simulink model "simulink_experiments_LQ_kal"  (R2019b)
settings: Solver=ode1  StartTime=0.0  StopTime=inf  FixedStep=0.002  RelTol=1e-3  EnableMultiTasking=on
PostLoadFcn:
  | qc_set_target_type(getConfigSet(bdroot, 'QUARC Default Target Configuration'));
undefined symbols (not defined in the file): HIL, kalmf, Klqi_int, Klqi_state, qc_get_step_size
libraries: quarc_library x4
settings Model: SimulationMode=external  ExtModeTrigDuration=5000  Creator=CFulford  LastModifiedBy=Student
settings SolverCC: PositivePriorityOrder=on
settings DataIOCC: LimitDataPoints=on  SaveFormat=Array  SignalLoggingSaveFormat=ModelDataLogs  ReturnWorkspaceOutputs=off
settings OptimizationCC: ExpressionDepthLimit=2147483647  InitFltsAndDblsToZero=on  LifeSpan=inf
settings DebuggingCC: SaveWithParameterizedLinksMsg=none  UnderspecifiedInitializationDetection=Classic  MergeDetectMultiDrivingBlocksExec=none  SolverPrmCheckMsg=warning  MultiTaskDSMMsg=warning  MultiTaskCondExecSysMsg=none  FcnCallInpInsideContextMsg=warning  StateNameClashWarn=warning  SFUnexpectedBacktrackingDiag=warning  SFNoUnconditionalDefaultTransitionDiag=warning  SFExecutionAtInitializationDiag=none  ArithmeticOperatorsInVariantConditions=warning
settings HardwareCC: ProdBitPerPointer=32  ProdBitPerSizeT=32  ProdBitPerPtrDiffT=32  ProdLargestAtomicFloat=None  ProdIntDivRoundTo=Undefined  ProdEndianess=Unspecified  ProdWordSize=32  ProdHWDeviceType=32-bit Generic
settings ModelReferenceCC: PropagateSignalLabelsOutOfModel=off
settings SFSimCC: SimUseLocalCustomCode=off  CustomCodeUndefinedFunction=UseInterfaceOnly
settings RTWCC: Description=QUARC Win64 Target  SystemTargetFile=quarc_win64.tlc  TemplateMakefile=quarc_default_tmf  RTWUseLocalCustomCode=off
settings CodeAppCC: StateflowObjectComments=on
settings STFCustomTargetCC: TargetPreCompLibLocation=C:\PROGRA~3\QUARC\lib\2019b\win64\release  ConcurrentExecutionCompliant=on  GeneratePreprocessorConditionals=Disable all  CombineOutputUpdateFcns=on  CPPClassGenCompliant=on  SystemTargetFile=quarc_win64.tlc
settings GRTTargetCC: TargetPreCompLibLocation=C:\PROGRA~3\QUARC\lib\2019b\win64\release  TargetLangStandard=C89/C90 (ANSI)  ParMdlRefBuildCompliant=off  CompOptLevelCompliant=off  GeneratePreprocessorConditionals=Disable all  MatFileLogging=off  UseToolchainInfoCompliant=off  ExtMode=on  ExtModeMexFile=quarc_comm
settings ConfigComp: CovMetricSettings=dw  CovHtmlReporting=on  CovSaveCumulativeToWorkspaceVar=on  CovSaveSingleToWorkspaceVar=on  CovExternalEMLEnable=off  CovSFcnEnable=off

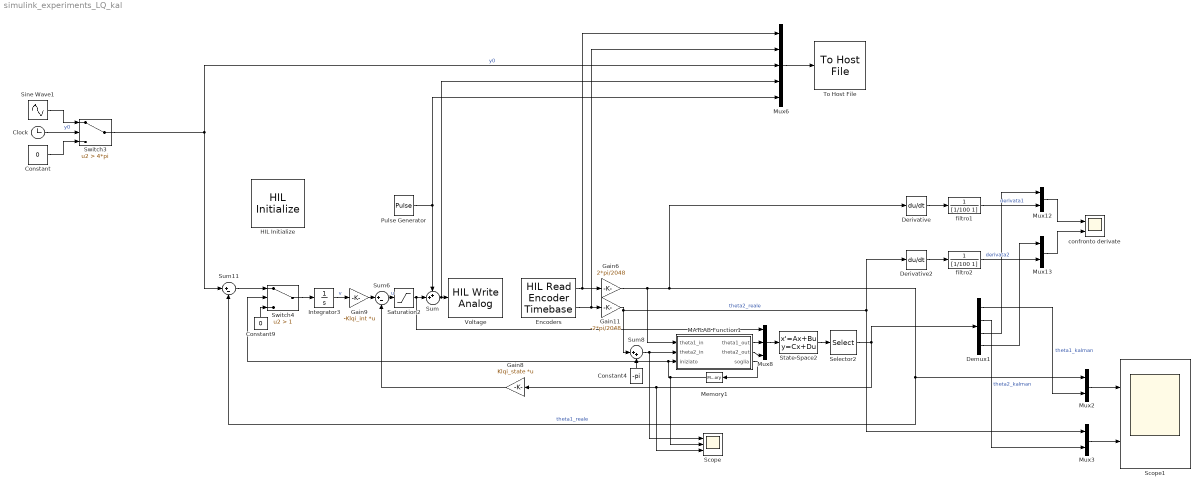
== system simulink_experiments_LQ_kal ==
  Clock : Clock
  Constant : Constant  Value=0
  Constant4 : Constant  Value=-pi
  Constant9 : Constant  Value=0
  Demux1 : Demux
  Derivative : Derivative
  Derivative2 : Derivative
  Encoders : quarc_library/Data Acquisition/Generic/Timebases/HIL Read Encoder Timebase  object_name=HIL-1  clock=0  channels=[0:1]  samples_in_buffer=max(ceil(1/qc_get_step_size), 1)  active=on  vector_output=off  data_type_mode=Inherit via back propagation  data_type=double
  Gain11 : Gain  Gain=-2*pi/2048
  Gain6 : Gain  Gain=2*pi/2048
  Gain8 : Gain  Gain=Klqi_state  Multiplication=Matrix(K*u)
  Gain9 : Gain  Gain=-Klqi_int  Multiplication=Matrix(K*u)
  HIL Initialize : quarc_library/Data Acquisition/Generic/Configuration/HIL Initialize  Priority=-99  object_name=HIL-1  board_type=qube_servo2_usb  board_number=0  board_options=""  exclusive=off  active=off  hardware_clocks=[0]  clock_modes=[]  initial_clock_frequencies=[]  set_clock_params_at_start=off  set_clock_params_at_switch_in=off  set_clock_frequencies_at_start=off  set_clock_frequencies_at_switch_in=off  analog_input_channels=[0]  analog_input_configurations=[]  analog_input_maximums=3  analog_input_minimums=-3  set_analog_input_params_at_start=off  set_analog_input_params_at_switch_in=off  analog_output_channels=[0]  analog_output_maximums=15  analog_output_minimums=-15  initial_analog_outputs=[0]  final_analog_outputs=[0]  watchdog_analog_outputs=0  set_analog_output_params_at_start=off  set_analog_output_params_at_switch_in=off  set_analog_outputs_at_start=on  set_analog_outputs_at_switch_in=off  set_analog_outputs_at_terminate=on  set_analog_outputs_at_switch_out=off  set_analog_outputs_on_watchdog=on  digital_input_channels=[]  digital_output_channels=[0]  digital_output_configuration=[]  initial_digital_outputs=[1]  final_digital_outputs=[0]  watchdog_digital_outputs=[0]  set_digital_output_params_at_start=off  set_digital_output_params_at_switch_in=off  set_digital_outputs_at_start=on  set_digital_outputs_at_switch_in=off  set_digital_outputs_at_terminate=on  set_digital_outputs_at_switch_out=off  set_digital_outputs_on_watchdog=on  encoder_channels=[0:1]  quadrature=[4]  encoder_filter_frequency=[]  initial_encoder_counts=[0]  set_encoder_params_at_start=off  set_encoder_params_at_switch_in=off  set_encoder_counts_at_start=on  set_encoder_counts_at_switch_in=off  pwm_channels=[]  pwm_modes=[]  pwm_frequency=[]  pwm_configuration=[]  pwm_alignment=[]  pwm_polarity=[]  pwm_leading_deadband=[]  pwm_trailing_deadband=[]  initial_pwm_outputs=[]  final_pwm_outputs=[]  watchdog_pwm_outputs=[]  set_pwm_params_at_start=off  set_pwm_params_at_switch_in=off  set_pwm_outputs_at_start=off  set_pwm_outputs_at_switch_in=off  set_pwm_outputs_at_terminate=off  set_pwm_outputs_at_switch_out=off  set_pwm_outputs_on_watchdog=off  other_output_channels=[11000:11002]  initial_other_outputs=[0 1 0]  final_other_outputs=[1 0 0]  watchdog_other_outputs=[0 0 1]  set_other_outputs_at_start=on  set_other_outputs_at_switch_in=off  set_other_outputs_at_terminate=on  set_other_outputs_at_switch_out=off  set_other_outputs_on_watchdog=on
  Integrator3 : Integrator
  MATLAB Function1 : MATLAB Function  TreatAsAtomicUnit=on
  Memory1 : Memory
  Mux{2..3,12..13} (4 alike) : Mux  Inputs=2
  Mux6 : Mux  Inputs=5
  Mux8 : Mux  Inputs=3
  Pulse Generator : DiscretePulseGenerator  PulseType=Time based  Amplitude=0.8  Period=10
  Saturation2 : Saturate  UpperLimit=10  LowerLimit=-10
  Scope : Scope  NumInputPorts=3
  Scope1 : Scope  NumInputPorts=2
  Selector2 : Selector  InputPortWidth=6  IndexOptions=Index vector (dialog)  Indices=[3,4,5,6]  OutputSizes=1
  Sine Wave1 : Sin  Amplitude=0  Frequency=30  SampleTime=0
  State-Space2 : StateSpace  A=kalmf.A  B=kalmf.B  C=kalmf.C  D=kalmf.D  InitialCondition=0
  Sum : Sum  Inputs=++|
  Sum11 : Sum  Inputs=|+-
  Sum6 : Sum  Inputs=|+-
  Sum8 : Sum  Inputs=|++
  Switch3 : Switch  Criteria=u2 > Threshold  Threshold=4*pi
  Switch4 : Switch  Criteria=u2 > Threshold  Threshold=1
  To Host File : quarc_library/Sinks/To Host/To Host File  file_name=data_%{date}_%{time}.mat  variable_name=data_%{date}_%{time}  decimation=1  sample_time=-1  file_format=MAT-file v.5  options=No header or footer  append=off  final_file_name=data_28-May-2024_18-36-20.mat  bitrate=2000000
  Voltage : quarc_library/Data Acquisition/Generic/Immediate I//O/HIL Write Analog  object_name=HIL-1  channels=0  sample_time=-1  active=off  vector_input=off
  "confronto derivate " : Scope  NumInputPorts=2
  filtro1 : TransferFcn  Denominator=[1/100 1]
  filtro2 : TransferFcn  Denominator=[1/100 1]
  wires:
  Derivative2/1 -> filtro2/1
  Mux13/1 -> "confronto derivate "/2
  State-Space2/1 -> Selector2/1
  Gain9/1 -> Sum6/1
  Gain11/1 -> Sum8/1, Mux3/1, Derivative2/1  "theta2_reale"
  Mux8/1 -> State-Space2/1
  Encoders/1 -> Gain6/1, Mux6/1
  Derivative/1 -> filtro1/1
  Constant4/1 -> Sum8/2
  filtro2/1 -> Mux13/2  "derivata2"
  Integrator3/1 -> Gain9/1  "v"
  Sum6/1 -> Saturation2/1  "u"
  Gain8/1 -> Sum6/2
  Encoders/2 -> Mux6/2, Gain11/1
  Mux6/1 -> To Host File/1
  Sum11/1 -> Switch4/1
  Memory1/1 -> Scope/2, Switch4/2, MATLAB Function1/3(iniziato)
  Selector2/1 -> Scope/3, Gain8/1, Demux1/1
  MATLAB Function1/1(theta1_out) -> Mux8/2
  MATLAB Function1/3(soglia) -> Memory1/1
  filtro1/1 -> Mux12/2  "derivata1"
  Sum8/1 -> Scope/1, MATLAB Function1/2(theta2_in)
  Mux12/1 -> "confronto derivate "/1
  MATLAB Function1/2(theta2_out) -> Mux8/3
  Constant9/1 -> Switch4/3
  Gain6/1 -> MATLAB Function1/1(theta1_in), Derivative/1, Mux2/1, Sum11/2  "theta1_reale"
  Switch4/1 -> Integrator3/1
  Saturation2/1 -> Mux8/1, Sum/2
  Sum/1 -> Mux6/4, Voltage/1
  Pulse Generator/1 -> Mux6/5, Sum/1
  Switch3/1 -> Sum11/1, Mux6/3  "y0"
  Demux1/3 -> Mux12/1
  Demux1/4 -> Mux13/1
  Demux1/1 -> Mux2/2  "theta1_kalman"
  Demux1/2 -> Mux3/2  "theta2_kalman"
  Mux2/1 -> Scope1/1
  Mux3/1 -> Scope1/2
  Sine Wave1/1 -> Switch3/1  "y0"
  Clock/1 -> Switch3/2
  Constant/1 -> Switch3/3

== matlab function simulink_experiments_LQ_kal/MATLAB Function1 ==
  data: theta1_in input; theta1_out output; theta2_in input; iniziato input double; theta2_out output; soglia output
function [theta1_out, theta2_out, soglia] = fcn(theta1_in, theta2_in, iniziato)
if theta2_in >= 0.01
    theta1_out = theta1_in;
    theta2_out = theta2_in;
    soglia = 2; 
elseif iniziato >1
    theta1_out = theta1_in;
    theta2_out = theta2_in;
    soglia = 2;
else
    soglia = 0;
    theta1_out = 0;
    theta2_out = 0;
end
% soglia = 2;s
% theta1_out = theta1_in;
% theta2_out = theta2_in;
end
